simulink model "buck"  (R2022b)
settings: Solver=FixedStepAuto  StartTime=0.0  StopTime=1  FixedStep=1e-6  MaxStep=1e-5  RelTol=1e-3
InitFcn:
  | clear all;
  | fs=1e4;
libraries: spsSeriesRLCBranchLib x3, spsCurrentMeasurementLib x1, spsDCVoltageSourceLib x1, spsDiodeLib x1, spsGroundLib x1, spsMosfetLib x1, simulink x1, spsVoltageMeasurementLib x1, sps_lib x1
settings Model: Creator=86135  LastModifiedBy=86135

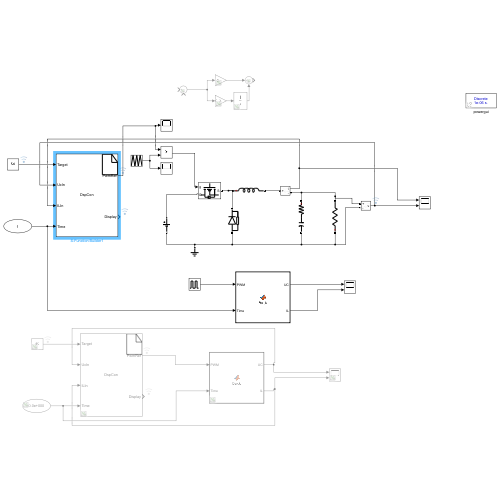
[thumbnail: Simulink's stored preview of the top-level diagram]
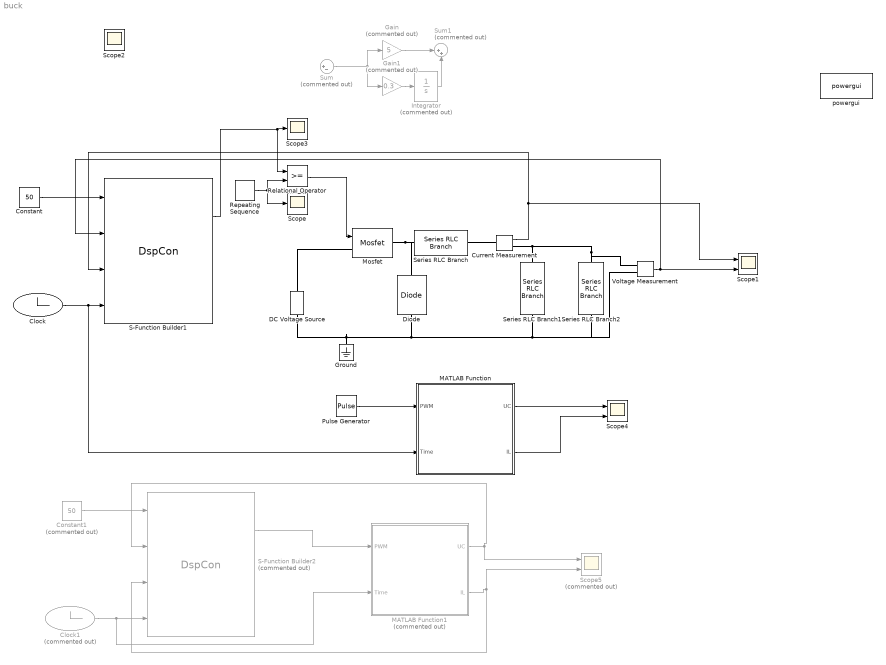
== system buck ==
  Clock : Clock
  Clock1 : Clock  Commented=on
  Constant : Constant  Value=50
  Constant1 : Constant  Commented=on  Value=50
  Current Measurement : spsCurrentMeasurementLib/Current Measurement  PhasorSimulation=off  OutputType=Complex  PSBequivalent=0
  DC Voltage Source : spsDCVoltageSourceLib/DC Voltage Source  Amplitude=100  Measurements=None
  Diode : spsDiodeLib/Diode  Ron=0.001  Lon=0  Vf=0.8  IC=0  UseSnubber=0  Rs=500  Cs=250e-9  Measurements=off
  Gain : Gain  Commented=on  Gain=5
  Gain1 : Gain  Commented=on  Gain=0.3
  Ground : spsGroundLib/Ground  LConnTagsString=a
  Integrator : Integrator  Commented=on
  MATLAB Function : MATLAB Function  TreatAsAtomicUnit=on
  MATLAB Function1 : MATLAB Function  Commented=on  TreatAsAtomicUnit=on
  Mosfet : spsMosfetLib/Mosfet  Ron=0.1  Lon=0  Rd=0.01  Vfd=0  IC=0  Rs=1e5  Cs=inf  Measurements=off
  Pulse Generator : DiscretePulseGenerator  PulseType=Time based  Period=1/10e4  PulseWidth=50
  Relational Operator : RelationalOperator  OutDataTypeStr=boolean  RndMeth=Simplest  InputSameDT=off
  Repeating Sequence : simulink/Sources/Repeating Sequence  rep_seq_t=[0 1/fs/2 1/fs]  rep_seq_y=[0 1 0]
  S-Function Builder1 : S-Function  FunctionName=DspCon  SFunctionModules=DspCon_wrapper.c ControlFunction BuckController  SFunctionDeploymentMode=off  EnableBusSupport=off  mask(S-Function Builder){}
      mask help: Simulink:masks:SFunctionBuilder_MD
      mask init:
      | val = [[.9  0.75 0.75 1 1 .9 .9 1]',[1 1 0.75 0.75 .9 .9 1 .9]'];try , sys = get_param(gcb,'SfunBuilderFcnName');if isempty(sys), sys = get_param(gcb,'FunctionName'); end,catch, sys = get_param(gcb,'FunctionName'); end
      settings: CopyFcn=set_param(gcbh,'LinkStatus','none')  PreSaveFcn=try, set_param(gcb,'FunctionName','DspCon'), end  OpenFcn=sfunctionwizard(gcbh)
      mask Display:
      | plot(val(:,1),val(:,2))
      | disp(sys)
      | port_label('input',1,'Target')
      | port_label('input',2,'UcIn')
      | port_label('input',3,'ILIn')
      | port_label('input',4,'Time')
      | port_label('output',1,'PwmRef')
      | port_label('output',2,'Display')
  S-Function Builder2 : S-Function  Commented=on  FunctionName=DspCon  SFunctionModules=DspCon_wrapper.c ControlFunction BuckController  SFunctionDeploymentMode=off  EnableBusSupport=off  mask(S-Function Builder){}
      mask help: Simulink:masks:SFunctionBuilder_MD
      mask init: same as buck/S-Function Builder1
      settings: CopyFcn=set_param(gcbh,'LinkStatus','none')  PreSaveFcn=try, set_param(gcb,'FunctionName','DspCon'), end  OpenFcn=sfunctionwizard(gcbh)
      mask Display:
      | plot(val(:,1),val(:,2))
      | disp(sys)
      | port_label('input',1,'Target')
      | port_label('input',2,'UcIn')
      | port_label('input',3,'ILIn')
      | port_label('input',4,'Time')
      | port_label('output',1,'PwmRef')
      | port_label('output',2,'Display')
  Scope : Scope
  Scope1 : Scope  NumInputPorts=2
  Scope3 : Scope
  Scope4 : Scope  NumInputPorts=2
  Scope5 : Scope  Commented=on  NumInputPorts=2
  Series RLC Branch : spsSeriesRLCBranchLib/Series RLC Branch  LConnTagsString=__new0  RConnTagsString=__new0  BranchType=L  Resistance=1  Inductance=1e-4  SetiL0=off  InitialCurrent=0  Capacitance=1e-6  Setx0=off  InitialVoltage=0  Measurements=None
  Series RLC Branch1 : spsSeriesRLCBranchLib/Series RLC Branch  LConnTagsString=__new0  RConnTagsString=__new0  BranchType=RC  Resistance=0.001  Inductance=1e-3  SetiL0=off  InitialCurrent=0  Capacitance=2200e-6  Setx0=off  InitialVoltage=0  Measurements=None
  Series RLC Branch2 : spsSeriesRLCBranchLib/Series RLC Branch  LConnTagsString=__new0  RConnTagsString=__new0  BranchType=R  Resistance=10  Inductance=1e-3  SetiL0=off  InitialCurrent=0  Capacitance=1e-6  Setx0=off  InitialVoltage=0  Measurements=None
  Sum : Sum  Commented=on  Inputs=|+-
  Sum1 : Sum  Commented=on  Inputs=|++
  Voltage Measurement : spsVoltageMeasurementLib/Voltage Measurement  PhasorSimulation=off  OutputType=Complex  PSBequivalent=0
  powergui : sps_lib/powergui  Priority=1  SimulationMode=Discrete  SampleTime=1e-6  frequency=60  Iterations=50  frequencyindice=0  Pbase=100e6  ErrMax=1e-4  UnitsV=kV  UnitsW=MW  buscounter=0  FunctionMessages=off  echomessages=off  EnableUseOfTLC=off  CurrentSourceSwitches=off  DisableSnubberDevices=off  DisableRonSwitches=off  DisableVfSwitches=off  DisplayEquations=off  AutomaticDiscreteSolvers=off  SolverType=Tustin/Backward Euler (TBE)  Interpol=off  ExternalGateDelay=off  methode=off  Ts=100  x0status=blocks  SPID=on  SwTol=0  HookPort=off  NonlinearTolerance=1e-4  nMaxIteration=100  ContinueOnMaxIteration=off  RestoreLinks=warning  ResistiveCurrentMeasurement=off  Frange=[0:2:500]  Ylog=off  Xlog=on  ShowGrid=off  save=off  variable=ZData  structure=0  ZoomFFT=off  StartTime=0.0  cycles=1  DisplayStyle=1  fundamental=60  FreqAxis=off  MaxFrequency=1000  frequencyindicesteady=1  RmsSteady=1  display=off
  Scope2 : Scope
  wires:
  Repeating Sequence/1 -> Scope/1, Relational Operator/2
  S-Function Builder1/1 -> Scope3/1, Relational Operator/1
  Voltage Measurement/1 -> S-Function Builder1/2, Scope1/2
  Constant/1 -> S-Function Builder1/1
  Gain/1 -> Sum1/1
  Sum/1 -> Gain1/1, Gain/1
  Integrator/1 -> Sum1/2
  Gain1/1 -> Integrator/1
  Clock/1 -> MATLAB Function/2(Time), S-Function Builder1/4
  Current Measurement/1 -> Scope1/1, S-Function Builder1/3
  MATLAB Function/1(UC) -> Scope4/1
  MATLAB Function/2(IL) -> Scope4/2
  Relational Operator/1 -> Mosfet/1
  S-Function Builder2/1 -> MATLAB Function1/1(PWM)
  Clock1/1 -> MATLAB Function1/2(Time), S-Function Builder2/4
  MATLAB Function1/1(UC) -> S-Function Builder2/2, Scope5/1
  MATLAB Function1/2(IL) -> Scope5/2, S-Function Builder2/3
  Constant1/1 -> S-Function Builder2/1
  Pulse Generator/1 -> MATLAB Function/1(PWM)
  connections:
  DC Voltage Source/RConn1 -- Mosfet/LConn1
  Diode/RConn1 -- Series RLC Branch/LConn1 -- Mosfet/RConn1
  Ground/LConn1 -- Voltage Measurement/LConn2 -- Series RLC Branch2/LConn1 -- Series RLC Branch1/RConn1 -- Diode/LConn1 -- DC Voltage Source/LConn1
  Series RLC Branch2/RConn1 -- Voltage Measurement/LConn1 -- Current Measurement/RConn1 -- Series RLC Branch1/LConn1
  Current Measurement/LConn1 -- Series RLC Branch/RConn1

== matlab function buck/MATLAB Function ==
  data: PWM input; UC output; Time input; IL output
function [UC,IL] = Buck(PWM,Time )
persistent IL_UC;

if  isempty(IL_UC)
    IL_UC = zeros(2,1);
end

persistent counter;

if isempty(counter)
    counter = zeros(1,1);
end

Ts = 1e-6;
C = 1e-5;
L = 1e-3;
R = 2;
Vg = 100;


if Time>counter*Ts
    
    counter = counter + 1;
    AA=[1 -Ts/L;Ts/C 1-Ts/(R*C)];
    BB=[Ts*Vg/L 0; 0 0];
    UU=[PWM;0];
    IL_UC=AA*IL_UC+BB*UU;
end

IL=IL_UC(1,1);
UC=IL_UC(2,1);

== matlab function buck/MATLAB Function1 ==
  data: PWM input; UC output; Time input; IL output
function [UC,IL] = Buck(PWM,Time )
persistent IL_UC;

if  isempty(IL_UC)
    IL_UC = zeros(2,1);
end

persistent counter;
if isempty(counter)
    counter = zeros(1,1);
end

Ts = 1e-6;
C = 1e-5;
L = 1e-3;
R = 2;
Vg = 100;


if Time>counter*Ts
    
    counter = counter + 1;
    AA=[1 -Ts/L;Ts/C 1-Ts/(R*C)];
    BB=[Ts*Vg/L 0; 0 0];
    UU=[PWM;0];
    IL_UC=AA*IL_UC+BB*UU;
end

IL=IL_UC(1,1);
UC=IL_UC(2,1);
